simulink model "mpc_nlm1"  (R2018a)
settings: Solver=ode45  StartTime=0.0  StopTime=10.0  RelTol=1e-3
settings Model: ExtModeTrigMode=oneshot  Creator=The MathWorks, Inc.  LastModifiedBy=Nakul
settings DataIOCC: SaveFormat=Array
settings OptimizationCC: BlockReduction=off  BooleanDataType=off  ExpressionDepthLimit=2147483647  LifeSpan=inf
settings DebuggingCC: SaveWithParameterizedLinksMsg=none  UnderspecifiedInitializationDetection=Classic  MergeDetectMultiDrivingBlocksExec=none  SignalResolutionControl=TryResolveAllWithWarning  MultiTaskDSMMsg=warning  MultiTaskCondExecSysMsg=none  FcnCallInpInsideContextMsg=warning  StateNameClashWarn=warning  SFUnexpectedBacktrackingDiag=warning  SFNoUnconditionalDefaultTransitionDiag=warning  SFExecutionAtInitializationDiag=none
settings HardwareCC: ProdBitPerPointer=32  ProdBitPerSizeT=32  ProdBitPerPtrDiffT=32  ProdLargestAtomicFloat=None  ProdIntDivRoundTo=Undefined  ProdEndianess=Unspecified  ProdWordSize=32  ProdHWDeviceType=32-bit Generic  TargetUnknown=on
settings ModelReferenceCC: PropagateSignalLabelsOutOfModel=off
settings CodeAppCC: StateflowObjectComments=on
settings GRTTargetCC: TargetLangStandard=C89/C90 (ANSI)  GeneratePreprocessorConditionals=Disable all  CombineOutputUpdateFcns=off  GRTInterface=on
settings ConfigComp: CovMetricSettings=dw  CovHtmlReporting=on  CovSaveCumulativeToWorkspaceVar=on  CovSaveSingleToWorkspaceVar=on  CovExternalEMLEnable=off  CovSFcnEnable=off

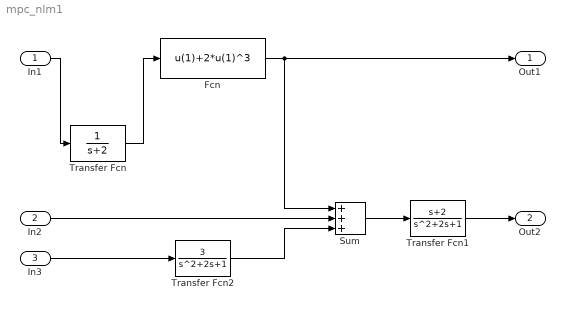
== system mpc_nlm1 ==
  In1 : Inport
  In2 : Inport  Port=2
  In3 : Inport  Port=3
  Fcn : Fcn  Expr=u(1)+2*u(1)^3
  Sum : Sum  Inputs=+++  SaturateOnIntegerOverflow=on  InputSameDT=on  OutDataTypeStr=Inherit: Same as first input
  Transfer Fcn : TransferFcn  Denominator=[1 2]
  Transfer Fcn1 : TransferFcn  Numerator=[1 2]
  Transfer Fcn2 : TransferFcn  Numerator=[3]
  Out1 : Outport
  Out2 : Outport  Port=2
  wires:
  In1/1 -> Transfer Fcn/1
  In3/1 -> Transfer Fcn2/1
  Transfer Fcn2/1 -> Sum/3
  Transfer Fcn/1 -> Fcn/1
  Fcn/1 -> Out1/1, Sum/1
  In2/1 -> Sum/2
  Transfer Fcn1/1 -> Out2/1
  Sum/1 -> Transfer Fcn1/1
